simulink model "QAM16"  (R2024a)
settings: Solver=ode45  StartTime=0.0  StopTime=5000  RelTol=1e-3  EnableMultiTasking=on
PreLoadFcn:
  | QAM16_PreLoadFcn
values from neighbouring files (symbols this model uses):
  chan = [1+j*0.1 .2 j*0.2 0 0 0 0 0 0 0]    [QAM16_PreLoadFcn.m]
  hh = sinc(-3:.25:3)    [QAM16_PreLoadFcn.m]
  k = 9    [QAM16_PreLoadFcn.m]
  k_i0 = (4*theta_0*theta_0)/(1+2*eta*theta_0+theta_0*theta_0)    [QAM16_PreLoadFcn.m]
  k_p0 = (4*eta*theta_0)/(1+2*eta*theta_0+theta_0*theta_0)    [QAM16_PreLoadFcn.m]
  mu = 0.004    [QAM16_PreLoadFcn.m]
undefined symbols (not defined in the file or in its folder): j, QAM, S, vsva2197, xcvc1902, xlipgetpartsetting
libraries: hdlBasic x260, dspmlti4 x2, hdlUtilities x1, hdlDSPIP x1, simulink x1, vmcUtilities x1
(part 3 of 3)

== system QAM16/DUT/Adaptive Equalizer/ALU/PE0/LMS Update/cb0 ==
  In : Inport
  Addressable Shift Register : hdlBasic/Addressable Shift Register  infer_latency=on  depth=2  initVector=[0 0 0]  en=on  use_behavioral_HDL=off  Optimization=Resource  use_rpm=off  XmcBlockStatus=1  maskContainerNames=group1  block_type=addrsr  block_config=sysgen:Addrsr_config
  Constant : hdlBasic/Constant  const=2  gui_display_data_type=Fixed-point  arith_type=Unsigned  n_bits=2  bin_pt=0  preci_type=Single  exp_width=8  frac_width=24  explicit_period=off  period=1  XmcBlockStatus=1  maskContainerNames=tabcontainer1  block_type=constant  block_config=sysgen:Constant_config
  Delay : hdlBasic/Delay  rst=off  en=off  latency=2  reg_retiming=off  XmcBlockStatus=1  maskContainerNames=group1  block_type=delay  block_config=sysgen:Delay_config
  F1 : hdlBasic/Relational  mode=a=b  op_type=Bool  en=off  latency=0  XmcBlockStatus=1  maskContainerNames=tabcontainer1  block_type=relational  block_config=sysgen:Relational_config
  Inverter : hdlBasic/Inverter  en=off  latency=0  XmcBlockStatus=1  maskContainerNames=group2  block_type=inv  block_config=sysgen:Inverter_config
  K1 : hdlBasic/Constant  const=0  gui_display_data_type=Fixed-point  arith_type=Unsigned  n_bits=7  bin_pt=0  preci_type=Single  exp_width=8  frac_width=24  explicit_period=on  period=T  XmcBlockStatus=1  maskContainerNames=tabcontainer1  block_type=constant  block_config=sysgen:Constant_config
  R5 : hdlBasic/Register  init=0  rst=off  en=on  XmcBlockStatus=1  maskContainerNames=tabcontainer1  block_type=register  block_config=sysgen:Register_config
  Startup Counter : hdlBasic/Counter  cnt_type=Count limited  cnt_to=0  operation=Down  start_count=60  cnt_by_val=1  arith_type=Unsigned  n_bits=7  bin_pt=0  load_pin=off  rst=off  en=on  explicit_period=Inferred from inputs  period=T  use_behavioral_HDL=off  implementation=Fabric  use_rpm=off  XmcBlockStatus=1  maskContainerNames=group1  block_type=counter  block_config=sysgen:Counter_config  block_width=531  block_height=1023
  Out : Outport  VectorParamsAs1DForOutWhenUnconnected=off
  wires:
  Addressable Shift Register/1 -> R5/1
  Delay/1 -> R5/2, Addressable Shift Register/3
  Constant/1 -> Addressable Shift Register/2
  Inverter/1 -> Startup Counter/1
  F1/1 -> Delay/1, Inverter/1
  In/1 -> Addressable Shift Register/1
  Startup Counter/1 -> F1/1
  K1/1 -> F1/2
  R5/1 -> Out/1

== system QAM16/DUT/Adaptive Equalizer/ALU/PE0/LMS Update/cb1 ==
  In : Inport
  Addressable Shift Register : hdlBasic/Addressable Shift Register  infer_latency=on  depth=2  initVector=[0 0 0]  en=on  use_behavioral_HDL=off  Optimization=Resource  use_rpm=off  XmcBlockStatus=1  maskContainerNames=group1  block_type=addrsr  block_config=sysgen:Addrsr_config
  Constant : hdlBasic/Constant  const=2  gui_display_data_type=Fixed-point  arith_type=Unsigned  n_bits=2  bin_pt=0  preci_type=Single  exp_width=8  frac_width=24  explicit_period=off  period=1  XmcBlockStatus=1  maskContainerNames=tabcontainer1  block_type=constant  block_config=sysgen:Constant_config
  Delay : hdlBasic/Delay  rst=off  en=off  latency=2  reg_retiming=off  XmcBlockStatus=1  maskContainerNames=group1  block_type=delay  block_config=sysgen:Delay_config
  F1 : hdlBasic/Relational  mode=a=b  op_type=Bool  en=off  latency=0  XmcBlockStatus=1  maskContainerNames=tabcontainer1  block_type=relational  block_config=sysgen:Relational_config
  Inverter : hdlBasic/Inverter  en=off  latency=0  XmcBlockStatus=1  maskContainerNames=group2  block_type=inv  block_config=sysgen:Inverter_config
  K1 : hdlBasic/Constant  const=0  gui_display_data_type=Fixed-point  arith_type=Unsigned  n_bits=7  bin_pt=0  preci_type=Single  exp_width=8  frac_width=24  explicit_period=on  period=T  XmcBlockStatus=1  maskContainerNames=tabcontainer1  block_type=constant  block_config=sysgen:Constant_config
  R5 : hdlBasic/Register  init=0  rst=off  en=on  XmcBlockStatus=1  maskContainerNames=tabcontainer1  block_type=register  block_config=sysgen:Register_config
  Startup Counter : hdlBasic/Counter  cnt_type=Count limited  cnt_to=0  operation=Down  start_count=60  cnt_by_val=1  arith_type=Unsigned  n_bits=7  bin_pt=0  load_pin=off  rst=off  en=on  explicit_period=Inferred from inputs  period=T  use_behavioral_HDL=off  implementation=Fabric  use_rpm=off  XmcBlockStatus=1  maskContainerNames=group1  block_type=counter  block_config=sysgen:Counter_config  block_width=531  block_height=1023
  Out : Outport  VectorParamsAs1DForOutWhenUnconnected=off
  wires:
  R5/1 -> Out/1
  K1/1 -> F1/2
  Startup Counter/1 -> F1/1
  In/1 -> Addressable Shift Register/1
  F1/1 -> Inverter/1, Delay/1
  Inverter/1 -> Startup Counter/1
  Constant/1 -> Addressable Shift Register/2
  Delay/1 -> Addressable Shift Register/3, R5/2
  Addressable Shift Register/1 -> R5/1

== system QAM16/DUT/Adaptive Equalizer/ALU/PE0/MAC FIR/Cmplx Mult ==
  a_r : Inport
  a_i : Inport  Port=2
  b_r : Inport  Port=3
  b_i : Inport  Port=4
  AddSub : hdlBasic/AddSub  mode=Addition  use_carryin=off  use_carryout=off  en=off  latency=1  precision=User Defined  arith_type="Signed  (2's comp)"  n_bits=lms_mult_post_add_ni  bin_pt=lms_mult_post_add_nf  quantization=Truncate  overflow=Wrap  use_behavioral_HDL=on  hw_selection=Fabric  pipelined=off  use_rpm=off  XmcBlockStatus=1  maskContainerNames=tabcontainer1  block_type=addsub  block_config=sysgen:Addsub_config
  AddSub1 : hdlBasic/AddSub  mode=Subtraction  use_carryin=off  use_carryout=off  en=off  latency=1  precision=User Defined  arith_type="Signed  (2's comp)"  n_bits=lms_mult_post_add_ni  bin_pt=lms_mult_post_add_nf  quantization=Truncate  overflow=Wrap  use_behavioral_HDL=on  hw_selection=Fabric  pipelined=off  use_rpm=off  XmcBlockStatus=1  maskContainerNames=tabcontainer1  block_type=addsub  block_config=sysgen:Addsub_config
  Mult{,1..3} (4 alike) : hdlBasic/Mult  precision=User Defined  arith_type="Signed  (2's comp)"  n_bits=lms_mult_ni  bin_pt=lms_mult_nf  quantization=Truncate  overflow=Wrap  en=off  latency=1  opt_float=off  fp_mult_usage=No Usage  use_behavioral_HDL=off  opt=Speed  use_embedded=on  optimum_pipeline=off  pipeline=off  use_rpm=off  placement_style=Rectangular shape  XmcBlockStatus=1  maskContainerNames=group1  block_type=mult  block_config=sysgen:Mult_config  block_width=598  block_height=876
  p_r : Outport  VectorParamsAs1DForOutWhenUnconnected=off
  p_i : Outport  Port=2  VectorParamsAs1DForOutWhenUnconnected=off
  wires:
  Mult2/1 -> AddSub1/2
  Mult3/1 -> AddSub1/1
  a_i/1 -> Mult1/1, Mult3/2
  b_r/1 -> Mult/2, Mult3/1
  b_i/1 -> Mult1/2, Mult2/2
  a_r/1 -> Mult/1, Mult2/1
  Mult/1 -> AddSub/1
  Mult1/1 -> AddSub/2
  AddSub/1 -> p_r/1
  AddSub1/1 -> p_i/1

== system QAM16/DUT/Adaptive Equalizer/ALU/PE1/LMS Update/Cmplx Mult ==
  a_r : Inport
  a_i : Inport  Port=2
  b_r : Inport  Port=3
  b_i : Inport  Port=4
  AddSub : hdlBasic/AddSub  mode=Subtraction  use_carryin=off  use_carryout=off  en=off  latency=1  precision=User Defined  arith_type="Signed  (2's comp)"  n_bits=lms_mult_post_add_ni  bin_pt=lms_mult_post_add_nf  quantization=Truncate  overflow=Wrap  use_behavioral_HDL=on  hw_selection=Fabric  pipelined=off  use_rpm=on  XmcBlockStatus=1  maskContainerNames=tabcontainer1  block_type=addsub  block_config=sysgen:Addsub_config
  AddSub1 : hdlBasic/AddSub  mode=Addition  use_carryin=off  use_carryout=off  en=off  latency=1  precision=User Defined  arith_type="Signed  (2's comp)"  n_bits=lms_mult_post_add_ni  bin_pt=lms_mult_post_add_nf  quantization=Truncate  overflow=Wrap  use_behavioral_HDL=on  hw_selection=Fabric  pipelined=off  use_rpm=on  XmcBlockStatus=1  maskContainerNames=tabcontainer1  block_type=addsub  block_config=sysgen:Addsub_config
  Mult{1..4} (4 alike) : hdlBasic/Mult  precision=User Defined  arith_type="Signed  (2's comp)"  n_bits=lms_mult_ni  bin_pt=lms_mult_nf  quantization=Truncate  overflow=Wrap  en=off  latency=1  opt_float=off  fp_mult_usage=No Usage  use_behavioral_HDL=off  opt=Speed  use_embedded=on  optimum_pipeline=off  pipeline=off  use_rpm=on  placement_style=Rectangular shape  XmcBlockStatus=1  maskContainerNames=group1  block_type=mult  block_config=sysgen:Mult_config  block_width=598  block_height=876
  p_r : Outport  VectorParamsAs1DForOutWhenUnconnected=off
  p_i : Outport  Port=2  VectorParamsAs1DForOutWhenUnconnected=off
  wires:
  AddSub1/1 -> p_i/1
  AddSub/1 -> p_r/1
  Mult3/1 -> AddSub1/2
  Mult2/1 -> AddSub1/1
  Mult1/1 -> AddSub/2
  a_r/1 -> Mult2/1, Mult4/1
  b_i/1 -> Mult2/2, Mult1/2
  b_r/1 -> Mult3/1, Mult4/2
  a_i/1 -> Mult3/2, Mult1/1
  Mult4/1 -> AddSub/1

== system QAM16/DUT/Adaptive Equalizer/ALU/PE1/LMS Update/Coeff Buffer1 ==
  In : Inport
  Addressable Shift Register : hdlBasic/Addressable Shift Register  infer_latency=on  depth=2  initVector=[0 0 1]  en=on  use_behavioral_HDL=off  Optimization=Resource  use_rpm=off  XmcBlockStatus=1  maskContainerNames=group1  block_type=addrsr  block_config=sysgen:Addrsr_config
  Constant : hdlBasic/Constant  const=2  gui_display_data_type=Fixed-point  arith_type=Unsigned  n_bits=2  bin_pt=0  preci_type=Single  exp_width=8  frac_width=24  explicit_period=off  period=1  XmcBlockStatus=1  maskContainerNames=tabcontainer1  block_type=constant  block_config=sysgen:Constant_config
  Delay : hdlBasic/Delay  rst=off  en=off  latency=2  reg_retiming=off  XmcBlockStatus=1  maskContainerNames=group1  block_type=delay  block_config=sysgen:Delay_config
  F1 : hdlBasic/Relational  mode=a=b  op_type=Bool  en=off  latency=0  XmcBlockStatus=1  maskContainerNames=tabcontainer1  block_type=relational  block_config=sysgen:Relational_config
  Inverter : hdlBasic/Inverter  en=off  latency=0  XmcBlockStatus=1  maskContainerNames=group2  block_type=inv  block_config=sysgen:Inverter_config
  K1 : hdlBasic/Constant  const=0  gui_display_data_type=Fixed-point  arith_type=Unsigned  n_bits=7  bin_pt=0  preci_type=Single  exp_width=8  frac_width=24  explicit_period=on  period=T  XmcBlockStatus=1  maskContainerNames=tabcontainer1  block_type=constant  block_config=sysgen:Constant_config
  R5 : hdlBasic/Register  init=0  rst=off  en=on  XmcBlockStatus=1  maskContainerNames=tabcontainer1  block_type=register  block_config=sysgen:Register_config
  Startup Counter : hdlBasic/Counter  cnt_type=Count limited  cnt_to=0  operation=Down  start_count=60  cnt_by_val=1  arith_type=Unsigned  n_bits=7  bin_pt=0  load_pin=off  rst=off  en=on  explicit_period=Inferred from inputs  period=T  use_behavioral_HDL=off  implementation=Fabric  use_rpm=off  XmcBlockStatus=1  maskContainerNames=group1  block_type=counter  block_config=sysgen:Counter_config  block_width=531  block_height=1023
  Out : Outport  VectorParamsAs1DForOutWhenUnconnected=off
  wires:
  R5/1 -> Out/1
  K1/1 -> F1/2
  Startup Counter/1 -> F1/1
  In/1 -> Addressable Shift Register/1
  F1/1 -> Inverter/1, Delay/1
  Inverter/1 -> Startup Counter/1
  Constant/1 -> Addressable Shift Register/2
  Delay/1 -> Addressable Shift Register/3, R5/2
  Addressable Shift Register/1 -> R5/1

== system QAM16/DUT/Adaptive Equalizer/ALU/PE1/LMS Update/Coeff Buffer2 ==
  In : Inport
  Addressable Shift Register : hdlBasic/Addressable Shift Register  infer_latency=on  depth=2  initVector=[0 0 0]  en=on  use_behavioral_HDL=off  Optimization=Resource  use_rpm=off  XmcBlockStatus=1  maskContainerNames=group1  block_type=addrsr  block_config=sysgen:Addrsr_config
  Constant : hdlBasic/Constant  const=2  gui_display_data_type=Fixed-point  arith_type=Unsigned  n_bits=2  bin_pt=0  preci_type=Single  exp_width=8  frac_width=24  explicit_period=off  period=1  XmcBlockStatus=1  maskContainerNames=tabcontainer1  block_type=constant  block_config=sysgen:Constant_config
  Delay : hdlBasic/Delay  rst=off  en=off  latency=2  reg_retiming=off  XmcBlockStatus=1  maskContainerNames=group1  block_type=delay  block_config=sysgen:Delay_config
  F1 : hdlBasic/Relational  mode=a=b  op_type=Bool  en=off  latency=0  XmcBlockStatus=1  maskContainerNames=tabcontainer1  block_type=relational  block_config=sysgen:Relational_config
  Inverter : hdlBasic/Inverter  en=off  latency=0  XmcBlockStatus=1  maskContainerNames=group2  block_type=inv  block_config=sysgen:Inverter_config
  K1 : hdlBasic/Constant  const=0  gui_display_data_type=Fixed-point  arith_type=Unsigned  n_bits=7  bin_pt=0  preci_type=Single  exp_width=8  frac_width=24  explicit_period=on  period=T  XmcBlockStatus=1  maskContainerNames=tabcontainer1  block_type=constant  block_config=sysgen:Constant_config
  R5 : hdlBasic/Register  init=0  rst=off  en=on  XmcBlockStatus=1  maskContainerNames=tabcontainer1  block_type=register  block_config=sysgen:Register_config
  Startup Counter : hdlBasic/Counter  cnt_type=Count limited  cnt_to=0  operation=Down  start_count=60  cnt_by_val=1  arith_type=Unsigned  n_bits=7  bin_pt=0  load_pin=off  rst=off  en=on  explicit_period=Inferred from inputs  period=T  use_behavioral_HDL=off  implementation=Fabric  use_rpm=off  XmcBlockStatus=1  maskContainerNames=group1  block_type=counter  block_config=sysgen:Counter_config  block_width=531  block_height=1023
  Out : Outport  VectorParamsAs1DForOutWhenUnconnected=off
  wires:
  Addressable Shift Register/1 -> R5/1
  Delay/1 -> R5/2, Addressable Shift Register/3
  Constant/1 -> Addressable Shift Register/2
  Inverter/1 -> Startup Counter/1
  F1/1 -> Delay/1, Inverter/1
  In/1 -> Addressable Shift Register/1
  Startup Counter/1 -> F1/1
  K1/1 -> F1/2
  R5/1 -> Out/1

== system QAM16/DUT/Adaptive Equalizer/ALU/PE1/MAC FIR/Cmplx Mult ==
  a_r : Inport
  a_i : Inport  Port=2
  b_r : Inport  Port=3
  b_i : Inport  Port=4
  AddSub : hdlBasic/AddSub  mode=Addition  use_carryin=off  use_carryout=off  en=off  latency=1  precision=User Defined  arith_type="Signed  (2's comp)"  n_bits=lms_mult_post_add_ni  bin_pt=lms_mult_post_add_nf  quantization=Truncate  overflow=Wrap  use_behavioral_HDL=on  hw_selection=Fabric  pipelined=off  use_rpm=off  XmcBlockStatus=1  maskContainerNames=tabcontainer1  block_type=addsub  block_config=sysgen:Addsub_config
  AddSub1 : hdlBasic/AddSub  mode=Subtraction  use_carryin=off  use_carryout=off  en=off  latency=1  precision=User Defined  arith_type="Signed  (2's comp)"  n_bits=lms_mult_post_add_ni  bin_pt=lms_mult_post_add_nf  quantization=Truncate  overflow=Wrap  use_behavioral_HDL=on  hw_selection=Fabric  pipelined=off  use_rpm=off  XmcBlockStatus=1  maskContainerNames=tabcontainer1  block_type=addsub  block_config=sysgen:Addsub_config
  Mult{,1..3} (4 alike) : hdlBasic/Mult  precision=User Defined  arith_type="Signed  (2's comp)"  n_bits=lms_mult_ni  bin_pt=lms_mult_nf  quantization=Truncate  overflow=Wrap  en=off  latency=1  opt_float=off  fp_mult_usage=No Usage  use_behavioral_HDL=off  opt=Speed  use_embedded=on  optimum_pipeline=off  pipeline=off  use_rpm=off  placement_style=Rectangular shape  XmcBlockStatus=1  maskContainerNames=group1  block_type=mult  block_config=sysgen:Mult_config  block_width=598  block_height=876
  p_r : Outport  VectorParamsAs1DForOutWhenUnconnected=off
  p_i : Outport  Port=2  VectorParamsAs1DForOutWhenUnconnected=off
  wires:
  Mult2/1 -> AddSub1/2
  Mult3/1 -> AddSub1/1
  a_i/1 -> Mult1/1, Mult3/2
  b_r/1 -> Mult/2, Mult3/1
  b_i/1 -> Mult1/2, Mult2/2
  a_r/1 -> Mult/1, Mult2/1
  Mult/1 -> AddSub/1
  Mult1/1 -> AddSub/2
  AddSub/1 -> p_r/1
  AddSub1/1 -> p_i/1

== system QAM16/DUT/Carrier Recovery/Phase Detector/Cordic/Cordic Fine Angle PE/Cordic PE0 ==
  x_n-1 : Inport
  y_n-1 : Inport  Port=2
  z_n-1 : Inport  Port=3
  AddSub : hdlBasic/AddSub  mode=Addition or Subtraction  use_carryin=off  use_carryout=off  en=off  latency=0  precision=Full  arith_type="Signed  (2's comp)"  n_bits=cordic_pe_nbits_total  bin_pt=cordic_pe_nbits_frac  quantization=Truncate  overflow=Wrap  use_behavioral_HDL=on  hw_selection=Fabric  pipelined=off  use_rpm=off  XmcBlockStatus=1  maskContainerNames=tabcontainer1  block_type=addsub  block_config=sysgen:Addsub_config
  AddSub1 : hdlBasic/AddSub  mode=Addition or Subtraction  use_carryin=off  use_carryout=off  en=off  latency=0  precision=Full  arith_type="Signed  (2's comp)"  n_bits=cordic_pe_nbits_total  bin_pt=cordic_pe_nbits_frac  quantization=Truncate  overflow=Wrap  use_behavioral_HDL=on  hw_selection=Fabric  pipelined=off  use_rpm=off  XmcBlockStatus=1  maskContainerNames=tabcontainer1  block_type=addsub  block_config=sysgen:Addsub_config
  AddSub2 : hdlBasic/AddSub  mode=Addition or Subtraction  use_carryin=off  use_carryout=off  en=off  latency=0  precision=Full  arith_type="Signed  (2's comp)"  n_bits=atan_nbits  bin_pt=atan_nbits_frac  quantization=Truncate  overflow=Wrap  use_behavioral_HDL=on  hw_selection=Fabric  pipelined=off  use_rpm=off  XmcBlockStatus=1  maskContainerNames=tabcontainer1  block_type=addsub  block_config=sysgen:Addsub_config
  Inverter : hdlBasic/Inverter  en=off  latency=0  XmcBlockStatus=1  maskContainerNames=group2  block_type=inv  block_config=sysgen:Inverter_config
  K : hdlBasic/Constant  const=atan(1/2^0)  gui_display_data_type=Fixed-point  arith_type=Signed (2's comp)  n_bits=atan_nbits  bin_pt=atan_nbits_frac  preci_type=Single  exp_width=8  frac_width=24  explicit_period=off  period=1  XmcBlockStatus=1  maskContainerNames=tabcontainer1  block_type=constant  block_config=sysgen:Constant_config
  Shift : hdlBasic/Shift  shift_dir=Right  shift_bits=0  en=off  latency=0  precision=Full  arith_type="Signed  (2's comp)"  n_bits=cordic_pe_nbits_total  bin_pt=cordic_pe_nbits_frac  quantization=Truncate  overflow=Wrap  XmcBlockStatus=1  maskContainerNames=group2  block_type=shift  block_config=sysgen:Shift_config
  Shift1 : hdlBasic/Shift  shift_dir=Right  shift_bits=0  en=off  latency=0  precision=Full  arith_type="Signed  (2's comp)"  n_bits=cordic_pe_nbits_total  bin_pt=cordic_pe_nbits_frac  quantization=Truncate  overflow=Wrap  XmcBlockStatus=1  maskContainerNames=group2  block_type=shift  block_config=sysgen:Shift_config
  Slice : hdlBasic/Slice  nbits=1  boolean_output=on  mode=Upper Bit Location + Width  bit1=0  base1=MSB of Input  bit0=0  base0=LSB of Input  XmcBlockStatus=1  maskContainerNames=group1  block_type=slice  block_config=sysgen:Slice_config
  x : Outport  VectorParamsAs1DForOutWhenUnconnected=off
  y : Outport  Port=2  VectorParamsAs1DForOutWhenUnconnected=off
  z : Outport  Port=3  VectorParamsAs1DForOutWhenUnconnected=off
  wires:
  Shift1/1 -> AddSub1/2
  Shift/1 -> AddSub/2
  K/1 -> AddSub2/2
  Inverter/1 -> AddSub1/3
  Slice/1 -> Inverter/1, AddSub2/3, AddSub/3
  AddSub2/1 -> z/1
  AddSub1/1 -> y/1
  z_n-1/1 -> AddSub2/1
  AddSub/1 -> x/1
  y_n-1/1 -> Shift/1, AddSub1/1, Slice/1
  x_n-1/1 -> Shift1/1, AddSub/1

== system QAM16/DUT/Carrier Recovery/Phase Detector/Cordic/Cordic Fine Angle PE/Cordic PE1 ==
  x_n-1 : Inport
  y_n-1 : Inport  Port=2
  z_n-1 : Inport  Port=3
  AddSub : hdlBasic/AddSub  mode=Addition or Subtraction  use_carryin=off  use_carryout=off  en=off  latency=0  precision=Full  arith_type="Signed  (2's comp)"  n_bits=cordic_pe_nbits_total  bin_pt=cordic_pe_nbits_frac  quantization=Truncate  overflow=Wrap  use_behavioral_HDL=on  hw_selection=Fabric  pipelined=off  use_rpm=off  XmcBlockStatus=1  maskContainerNames=tabcontainer1  block_type=addsub  block_config=sysgen:Addsub_config
  AddSub1 : hdlBasic/AddSub  mode=Addition or Subtraction  use_carryin=off  use_carryout=off  en=off  latency=0  precision=Full  arith_type="Signed  (2's comp)"  n_bits=cordic_pe_nbits_total  bin_pt=cordic_pe_nbits_frac  quantization=Truncate  overflow=Wrap  use_behavioral_HDL=on  hw_selection=Fabric  pipelined=off  use_rpm=off  XmcBlockStatus=1  maskContainerNames=tabcontainer1  block_type=addsub  block_config=sysgen:Addsub_config
  AddSub2 : hdlBasic/AddSub  mode=Addition or Subtraction  use_carryin=off  use_carryout=off  en=off  latency=0  precision=Full  arith_type="Signed  (2's comp)"  n_bits=atan_nbits  bin_pt=atan_nbits_frac  quantization=Truncate  overflow=Wrap  use_behavioral_HDL=on  hw_selection=Fabric  pipelined=off  use_rpm=off  XmcBlockStatus=1  maskContainerNames=tabcontainer1  block_type=addsub  block_config=sysgen:Addsub_config
  Inverter : hdlBasic/Inverter  en=off  latency=0  XmcBlockStatus=1  maskContainerNames=group2  block_type=inv  block_config=sysgen:Inverter_config
  K : hdlBasic/Constant  const=atan(1/2^1)  gui_display_data_type=Fixed-point  arith_type=Signed (2's comp)  n_bits=atan_nbits  bin_pt=atan_nbits_frac  preci_type=Single  exp_width=8  frac_width=24  explicit_period=off  period=1  XmcBlockStatus=1  maskContainerNames=tabcontainer1  block_type=constant  block_config=sysgen:Constant_config
  Shift : hdlBasic/Shift  shift_dir=Right  shift_bits=1  en=off  latency=0  precision=Full  arith_type="Signed  (2's comp)"  n_bits=cordic_pe_nbits_total  bin_pt=cordic_pe_nbits_frac  quantization=Truncate  overflow=Wrap  XmcBlockStatus=1  maskContainerNames=group2  block_type=shift  block_config=sysgen:Shift_config
  Shift1 : hdlBasic/Shift  shift_dir=Right  shift_bits=1  en=off  latency=0  precision=Full  arith_type="Signed  (2's comp)"  n_bits=cordic_pe_nbits_total  bin_pt=cordic_pe_nbits_frac  quantization=Truncate  overflow=Wrap  XmcBlockStatus=1  maskContainerNames=group2  block_type=shift  block_config=sysgen:Shift_config
  Slice : hdlBasic/Slice  nbits=1  boolean_output=on  mode=Upper Bit Location + Width  bit1=0  base1=MSB of Input  bit0=0  base0=LSB of Input  XmcBlockStatus=1  maskContainerNames=group1  block_type=slice  block_config=sysgen:Slice_config
  x : Outport  VectorParamsAs1DForOutWhenUnconnected=off
  y : Outport  Port=2  VectorParamsAs1DForOutWhenUnconnected=off
  z : Outport  Port=3  VectorParamsAs1DForOutWhenUnconnected=off
  wires:
  x_n-1/1 -> AddSub/1, Shift1/1
  y_n-1/1 -> Slice/1, AddSub1/1, Shift/1
  AddSub/1 -> x/1
  z_n-1/1 -> AddSub2/1
  AddSub1/1 -> y/1
  AddSub2/1 -> z/1
  Slice/1 -> AddSub/3, AddSub2/3, Inverter/1
  Inverter/1 -> AddSub1/3
  K/1 -> AddSub2/2
  Shift/1 -> AddSub/2
  Shift1/1 -> AddSub1/2

== system QAM16/DUT/Carrier Recovery/Phase Detector/Cordic/Cordic Fine Angle PE/Cordic PE2 ==
  x_n-1 : Inport
  y_n-1 : Inport  Port=2
  z_n-1 : Inport  Port=3
  AddSub : hdlBasic/AddSub  mode=Addition or Subtraction  use_carryin=off  use_carryout=off  en=off  latency=0  precision=Full  arith_type="Signed  (2's comp)"  n_bits=cordic_pe_nbits_total  bin_pt=cordic_pe_nbits_frac  quantization=Truncate  overflow=Wrap  use_behavioral_HDL=on  hw_selection=Fabric  pipelined=off  use_rpm=off  XmcBlockStatus=1  maskContainerNames=tabcontainer1  block_type=addsub  block_config=sysgen:Addsub_config
  AddSub1 : hdlBasic/AddSub  mode=Addition or Subtraction  use_carryin=off  use_carryout=off  en=off  latency=0  precision=Full  arith_type="Signed  (2's comp)"  n_bits=cordic_pe_nbits_total  bin_pt=cordic_pe_nbits_frac  quantization=Truncate  overflow=Wrap  use_behavioral_HDL=on  hw_selection=Fabric  pipelined=off  use_rpm=off  XmcBlockStatus=1  maskContainerNames=tabcontainer1  block_type=addsub  block_config=sysgen:Addsub_config
  AddSub2 : hdlBasic/AddSub  mode=Addition or Subtraction  use_carryin=off  use_carryout=off  en=off  latency=0  precision=Full  arith_type="Signed  (2's comp)"  n_bits=atan_nbits  bin_pt=atan_nbits_frac  quantization=Truncate  overflow=Wrap  use_behavioral_HDL=on  hw_selection=Fabric  pipelined=off  use_rpm=off  XmcBlockStatus=1  maskContainerNames=tabcontainer1  block_type=addsub  block_config=sysgen:Addsub_config
  Inverter : hdlBasic/Inverter  en=off  latency=0  XmcBlockStatus=1  maskContainerNames=group2  block_type=inv  block_config=sysgen:Inverter_config
  K : hdlBasic/Constant  const=atan(1/2^2)  gui_display_data_type=Fixed-point  arith_type=Signed (2's comp)  n_bits=atan_nbits  bin_pt=atan_nbits_frac  preci_type=Single  exp_width=8  frac_width=24  explicit_period=off  period=1  XmcBlockStatus=1  maskContainerNames=tabcontainer1  block_type=constant  block_config=sysgen:Constant_config
  Shift : hdlBasic/Shift  shift_dir=Right  shift_bits=2  en=off  latency=0  precision=Full  arith_type="Signed  (2's comp)"  n_bits=cordic_pe_nbits_total  bin_pt=cordic_pe_nbits_frac  quantization=Truncate  overflow=Wrap  XmcBlockStatus=1  maskContainerNames=group2  block_type=shift  block_config=sysgen:Shift_config
  Shift1 : hdlBasic/Shift  shift_dir=Right  shift_bits=2  en=off  latency=0  precision=Full  arith_type="Signed  (2's comp)"  n_bits=cordic_pe_nbits_total  bin_pt=cordic_pe_nbits_frac  quantization=Truncate  overflow=Wrap  XmcBlockStatus=1  maskContainerNames=group2  block_type=shift  block_config=sysgen:Shift_config
  Slice : hdlBasic/Slice  nbits=1  boolean_output=on  mode=Upper Bit Location + Width  bit1=0  base1=MSB of Input  bit0=0  base0=LSB of Input  XmcBlockStatus=1  maskContainerNames=group1  block_type=slice  block_config=sysgen:Slice_config
  x : Outport  VectorParamsAs1DForOutWhenUnconnected=off
  y : Outport  Port=2  VectorParamsAs1DForOutWhenUnconnected=off
  z : Outport  Port=3  VectorParamsAs1DForOutWhenUnconnected=off
  wires:
  Shift1/1 -> AddSub1/2
  Shift/1 -> AddSub/2
  K/1 -> AddSub2/2
  Inverter/1 -> AddSub1/3
  Slice/1 -> Inverter/1, AddSub2/3, AddSub/3
  AddSub2/1 -> z/1
  AddSub1/1 -> y/1
  z_n-1/1 -> AddSub2/1
  AddSub/1 -> x/1
  y_n-1/1 -> Shift/1, AddSub1/1, Slice/1
  x_n-1/1 -> Shift1/1, AddSub/1

== system QAM16/DUT/Carrier Recovery/Phase Detector/Cordic/Cordic Fine Angle PE/Cordic PE3 ==
  x_n-1 : Inport
  y_n-1 : Inport  Port=2
  z_n-1 : Inport  Port=3
  AddSub : hdlBasic/AddSub  mode=Addition or Subtraction  use_carryin=off  use_carryout=off  en=off  latency=0  precision=Full  arith_type="Signed  (2's comp)"  n_bits=cordic_pe_nbits_total  bin_pt=cordic_pe_nbits_frac  quantization=Truncate  overflow=Wrap  use_behavioral_HDL=on  hw_selection=Fabric  pipelined=off  use_rpm=off  XmcBlockStatus=1  maskContainerNames=tabcontainer1  block_type=addsub  block_config=sysgen:Addsub_config
  AddSub1 : hdlBasic/AddSub  mode=Addition or Subtraction  use_carryin=off  use_carryout=off  en=off  latency=0  precision=Full  arith_type="Signed  (2's comp)"  n_bits=cordic_pe_nbits_total  bin_pt=cordic_pe_nbits_frac  quantization=Truncate  overflow=Wrap  use_behavioral_HDL=on  hw_selection=Fabric  pipelined=off  use_rpm=off  XmcBlockStatus=1  maskContainerNames=tabcontainer1  block_type=addsub  block_config=sysgen:Addsub_config
  AddSub2 : hdlBasic/AddSub  mode=Addition or Subtraction  use_carryin=off  use_carryout=off  en=off  latency=0  precision=Full  arith_type="Signed  (2's comp)"  n_bits=atan_nbits  bin_pt=atan_nbits_frac  quantization=Truncate  overflow=Wrap  use_behavioral_HDL=on  hw_selection=Fabric  pipelined=off  use_rpm=off  XmcBlockStatus=1  maskContainerNames=tabcontainer1  block_type=addsub  block_config=sysgen:Addsub_config
  Inverter : hdlBasic/Inverter  en=off  latency=0  XmcBlockStatus=1  maskContainerNames=group2  block_type=inv  block_config=sysgen:Inverter_config
  K : hdlBasic/Constant  const=atan(1/2^3)  gui_display_data_type=Fixed-point  arith_type=Signed (2's comp)  n_bits=atan_nbits  bin_pt=atan_nbits_frac  preci_type=Single  exp_width=8  frac_width=24  explicit_period=off  period=1  XmcBlockStatus=1  maskContainerNames=tabcontainer1  block_type=constant  block_config=sysgen:Constant_config
  Shift : hdlBasic/Shift  shift_dir=Right  shift_bits=3  en=off  latency=0  precision=Full  arith_type="Signed  (2's comp)"  n_bits=cordic_pe_nbits_total  bin_pt=cordic_pe_nbits_frac  quantization=Truncate  overflow=Wrap  XmcBlockStatus=1  maskContainerNames=group2  block_type=shift  block_config=sysgen:Shift_config
  Shift1 : hdlBasic/Shift  shift_dir=Right  shift_bits=3  en=off  latency=0  precision=Full  arith_type="Signed  (2's comp)"  n_bits=cordic_pe_nbits_total  bin_pt=cordic_pe_nbits_frac  quantization=Truncate  overflow=Wrap  XmcBlockStatus=1  maskContainerNames=group2  block_type=shift  block_config=sysgen:Shift_config
  Slice : hdlBasic/Slice  nbits=1  boolean_output=on  mode=Upper Bit Location + Width  bit1=0  base1=MSB of Input  bit0=0  base0=LSB of Input  XmcBlockStatus=1  maskContainerNames=group1  block_type=slice  block_config=sysgen:Slice_config
  x : Outport  VectorParamsAs1DForOutWhenUnconnected=off
  y : Outport  Port=2  VectorParamsAs1DForOutWhenUnconnected=off
  z : Outport  Port=3  VectorParamsAs1DForOutWhenUnconnected=off
  wires:
  x_n-1/1 -> AddSub/1, Shift1/1
  y_n-1/1 -> Slice/1, AddSub1/1, Shift/1
  AddSub/1 -> x/1
  z_n-1/1 -> AddSub2/1
  AddSub1/1 -> y/1
  AddSub2/1 -> z/1
  Slice/1 -> AddSub/3, AddSub2/3, Inverter/1
  Inverter/1 -> AddSub1/3
  K/1 -> AddSub2/2
  Shift/1 -> AddSub/2
  Shift1/1 -> AddSub1/2

== system QAM16/DUT/Carrier Recovery/Phase Detector/Cordic/Cordic Fine Angle PE/Cordic PE4 ==
  x_n-1 : Inport
  y_n-1 : Inport  Port=2
  z_n-1 : Inport  Port=3
  AddSub : hdlBasic/AddSub  mode=Addition or Subtraction  use_carryin=off  use_carryout=off  en=off  latency=0  precision=Full  arith_type="Signed  (2's comp)"  n_bits=cordic_pe_nbits_total  bin_pt=cordic_pe_nbits_frac  quantization=Truncate  overflow=Wrap  use_behavioral_HDL=on  hw_selection=Fabric  pipelined=off  use_rpm=off  XmcBlockStatus=1  maskContainerNames=tabcontainer1  block_type=addsub  block_config=sysgen:Addsub_config
  AddSub1 : hdlBasic/AddSub  mode=Addition or Subtraction  use_carryin=off  use_carryout=off  en=off  latency=0  precision=Full  arith_type="Signed  (2's comp)"  n_bits=cordic_pe_nbits_total  bin_pt=cordic_pe_nbits_frac  quantization=Truncate  overflow=Wrap  use_behavioral_HDL=on  hw_selection=Fabric  pipelined=off  use_rpm=off  XmcBlockStatus=1  maskContainerNames=tabcontainer1  block_type=addsub  block_config=sysgen:Addsub_config
  AddSub2 : hdlBasic/AddSub  mode=Addition or Subtraction  use_carryin=off  use_carryout=off  en=off  latency=0  precision=Full  arith_type="Signed  (2's comp)"  n_bits=atan_nbits  bin_pt=atan_nbits_frac  quantization=Truncate  overflow=Wrap  use_behavioral_HDL=on  hw_selection=Fabric  pipelined=off  use_rpm=off  XmcBlockStatus=1  maskContainerNames=tabcontainer1  block_type=addsub  block_config=sysgen:Addsub_config
  Inverter : hdlBasic/Inverter  en=off  latency=0  XmcBlockStatus=1  maskContainerNames=group2  block_type=inv  block_config=sysgen:Inverter_config
  K : hdlBasic/Constant  const=atan(1/2^4)  gui_display_data_type=Fixed-point  arith_type=Signed (2's comp)  n_bits=atan_nbits  bin_pt=atan_nbits_frac  preci_type=Single  exp_width=8  frac_width=24  explicit_period=off  period=1  XmcBlockStatus=1  maskContainerNames=tabcontainer1  block_type=constant  block_config=sysgen:Constant_config
  Shift : hdlBasic/Shift  shift_dir=Right  shift_bits=4  en=off  latency=0  precision=Full  arith_type="Signed  (2's comp)"  n_bits=cordic_pe_nbits_total  bin_pt=cordic_pe_nbits_frac  quantization=Truncate  overflow=Wrap  XmcBlockStatus=1  maskContainerNames=group2  block_type=shift  block_config=sysgen:Shift_config
  Shift1 : hdlBasic/Shift  shift_dir=Right  shift_bits=4  en=off  latency=0  precision=Full  arith_type="Signed  (2's comp)"  n_bits=cordic_pe_nbits_total  bin_pt=cordic_pe_nbits_frac  quantization=Truncate  overflow=Wrap  XmcBlockStatus=1  maskContainerNames=group2  block_type=shift  block_config=sysgen:Shift_config
  Slice : hdlBasic/Slice  nbits=1  boolean_output=on  mode=Upper Bit Location + Width  bit1=0  base1=MSB of Input  bit0=0  base0=LSB of Input  XmcBlockStatus=1  maskContainerNames=group1  block_type=slice  block_config=sysgen:Slice_config
  x : Outport  VectorParamsAs1DForOutWhenUnconnected=off
  y : Outport  Port=2  VectorParamsAs1DForOutWhenUnconnected=off
  z : Outport  Port=3  VectorParamsAs1DForOutWhenUnconnected=off
  wires:
  Shift1/1 -> AddSub1/2
  Shift/1 -> AddSub/2
  K/1 -> AddSub2/2
  Inverter/1 -> AddSub1/3
  Slice/1 -> Inverter/1, AddSub2/3, AddSub/3
  AddSub2/1 -> z/1
  AddSub1/1 -> y/1
  z_n-1/1 -> AddSub2/1
  AddSub/1 -> x/1
  y_n-1/1 -> Shift/1, AddSub1/1, Slice/1
  x_n-1/1 -> Shift1/1, AddSub/1
